simulink library "rotMat2Quat_ul"  (R2018b)
settings: Solver=VariableStepAuto  StartTime=0.0  StopTime=10.0  RelTol=1e-3
settings Model: Creator=mcobb  LastModifiedBy=mcobb

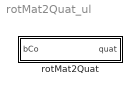
== system rotMat2Quat_ul ==
  rotMat2Quat : Subsystem

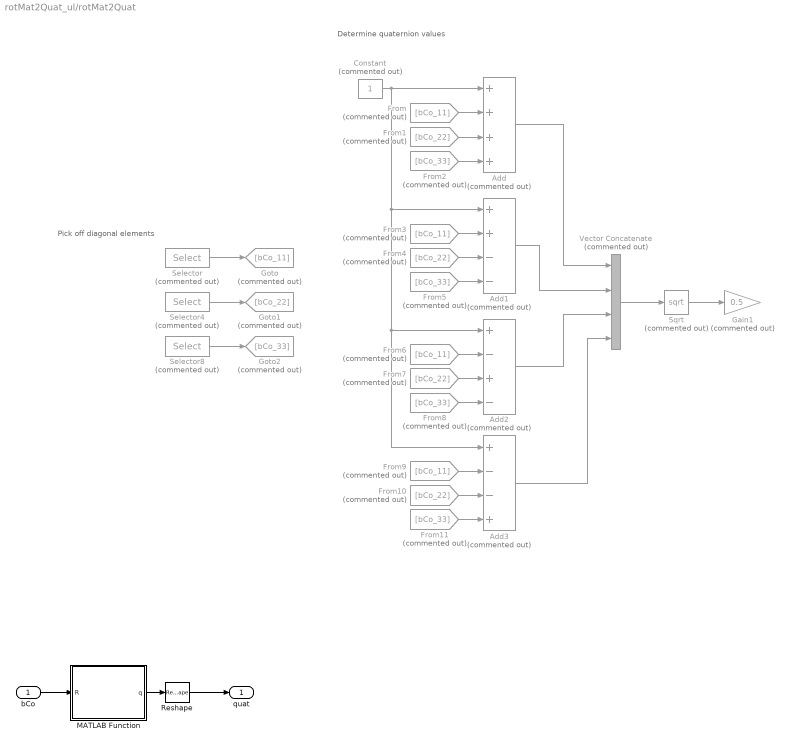
== system rotMat2Quat_ul/rotMat2Quat ==
  note: Pick off diagonal elements
  note: Determine quaternion values
  bCo : Inport
  Add : Sum  Commented=on  Inputs=++++
  Add1 : Sum  Commented=on  Inputs=++--
  Add2 : Sum  Commented=on  Inputs=+-+-
  Add3 : Sum  Commented=on  Inputs=+--+
  Constant : Constant  Commented=on
  From{,3,6,9} (4 alike) : From  Commented=on  GotoTag=bCo_11
  From{1,4,7,10} (4 alike) : From  Commented=on  GotoTag=bCo_22
  From{2,5,8,11} (4 alike) : From  Commented=on  GotoTag=bCo_33
  Gain1 : Gain  Commented=on  Gain=0.5
  Goto : Goto  Commented=on  GotoTag=bCo_11
  Goto1 : Goto  Commented=on  GotoTag=bCo_22
  Goto2 : Goto  Commented=on  GotoTag=bCo_33
  MATLAB Function : MATLAB Function  TreatAsAtomicUnit=on
  Reshape : Reshape  OutputDimensionality=Column vector (2-D)
  Selector : Selector  Commented=on  NumberOfDimensions=2  InputPortWidth=3  IndexOptions=Index vector (dialog),Index vector (dialog)  Indices=1,1  OutputSizes=1,1
  Selector4 : Selector  Commented=on  NumberOfDimensions=2  InputPortWidth=3  IndexOptions=Index vector (dialog),Index vector (dialog)  Indices=2,2  OutputSizes=1,1
  Selector8 : Selector  Commented=on  NumberOfDimensions=2  InputPortWidth=3  IndexOptions=Index vector (dialog),Index vector (dialog)  Indices=3,3  OutputSizes=1,1
  Sqrt : Sqrt  Commented=on  SaturateOnIntegerOverflow=on
  Vector Concatenate : Concatenate  Commented=on  NumInputs=4
  quat : Outport  PortDimensions=[4,1]
  wires:
  Selector/1 -> Goto/1
  Selector8/1 -> Goto2/1
  Selector4/1 -> Goto1/1
  From2/1 -> Add/4
  From1/1 -> Add/3
  From/1 -> Add/2
  Constant/1 -> Add3/1, Add2/1, Add1/1, Add/1
  From4/1 -> Add1/3
  From5/1 -> Add1/4
  From3/1 -> Add1/2
  From7/1 -> Add2/3
  From8/1 -> Add2/4
  From6/1 -> Add2/2
  From10/1 -> Add3/3
  From11/1 -> Add3/4
  From9/1 -> Add3/2
  Vector Concatenate/1 -> Sqrt/1
  Add/1 -> Vector Concatenate/1
  Add1/1 -> Vector Concatenate/2
  Add2/1 -> Vector Concatenate/3
  Add3/1 -> Vector Concatenate/4
  Sqrt/1 -> Gain1/1
  bCo/1 -> MATLAB Function/1(R)
  Reshape/1 -> quat/1
  MATLAB Function/1(q) -> Reshape/1

== matlab function rotMat2Quat_ul/rotMat2Quat/MATLAB Function ==
  data: R input; q output
function q = eulAng2Quat(R)
q = zeros(4,1);

% Extracting elements
R11 = R(1,1);
R12 = R(1,2);
R13 = R(1,3);
R21 = R(2,1);
R22 = R(2,2);
R23 = R(2,3);
R31 = R(3,1);
R32 = R(3,2);
R33 = R(3,3);

% Calculating squares elements
q0 = (1 + R11 + R22 + R33)/4;
q1 = (1 + R11 - R22 - R33)/4;
q2 = (1 - R11 + R22 - R33)/4;
q3 = (1 - R11 - R22 + R33)/4;

% qMag = sqrt(sum([q0 q1 q2 q3].^2));
% q0 = q0/qMag;
% q1 = q1/qMag;
% q2 = q2/qMag;
% q3 = q3/qMag;


% Choosing the max of the squares
[~,qIdx] = max([q0 q1 q2 q3]);

switch qIdx-1
    case 0
        q0 = sqrt(q0);
        q1 = (R32-R23)/(4*q0);
        q2 = (R13-R31)/(4*q0);
        q3 = (R21-R12)/(4*q0);
    case 1
        q1 = sqrt(q1);
        q0 = (R32-R23)/(4*q1);
        q2 = (R21+R12)/(4*q1);
        q3 = (R13+R31)/(4*q1);
    case 2
        q2 = sqrt(q2);
        q0 = (R13-R31)/(4*q2);
        q1 = (R21+R12)/(4*q2);
        q3 = (R32+R23)/(4*q2);
    case 3
        q3 = sqrt(q3);
        q0 = (R21-R12)/(4*q3);
        q1 = (R13+R31)/(4*q3);
        q2 = (R32+R23)/(4*q3);
end

q(1) = q0;
q(2) = q1;
q(3) = q2;
q(4) = q3;

q
sqrt(sum(q.^2,1))


% % Solving for quaternions
% if q_no == 1
%     q0 = sqrt(max_q);
%     
%     q1 = ((1/4)*(R32 - R23))/q0;
%     q2 = ((1/4)*(R13 - R31))/q0;
%     q3 = ((1/4)*(R21 - R12))/q0;
%     
% elseif q_no == 2
%     q1 = sqrt(max_q);
%     
%     q0 = ((1/4)*(R32 - R23))/q1;
%     q2 = ((1/4)*(R12 + R21))/q1;
%     q3 = ((1/4)*(R13 + R31))/q1;
%     
% elseif q_no == 3
%     q2 = sqrt(max_q);
%     
%     q0 = ((1/4)*(R13 - R31))/q2;
%     q1 = ((1/4)*(R12 + R21))/q2;
%     q3 = ((1/4)*(R23 + R32))/q2;
%     
% elseif q_no == 4
%     q3 = sqrt(max_q);
%     
%     q0 = ((1/4)*(R21 - R12))/q3;
%     q1 = ((1/4)*(R13 + R31))/q3;
%     q2 = ((1/4)*(R23 + R32))/q3;
%     
% end


end
